simulink model "LQR_control"  (R2020b)
settings: Solver=VariableStepAuto  StartTime=0.0  StopTime=180  RelTol=1e-3
values from neighbouring files (symbols this model uses):
  A_m = [0 1 0; M_alpha 0 M_alpha/V; -(F+N_alpha)/m 0 -N_alpha/(m*V)]    [state_space.m]
  B_m = [0;M_delta;Tc/m]    [state_space.m]
  C_m = diag([1 1 1])    [state_space.m]
  D_m = [0;0;0]    [state_space.m]
  K_1 = K(1)    [state_space.m]
  K_2 = K(2)    [state_space.m]
  K_3 = K(3)    [state_space.m]
  m = 38901    [state_space.m]
undefined symbols (not defined in the file or in its folder): Earth, WGS84
libraries: aerolibtransform2 x1, aerolibfltsims x1
settings Model: Creator=surya  LastModifiedBy=surya

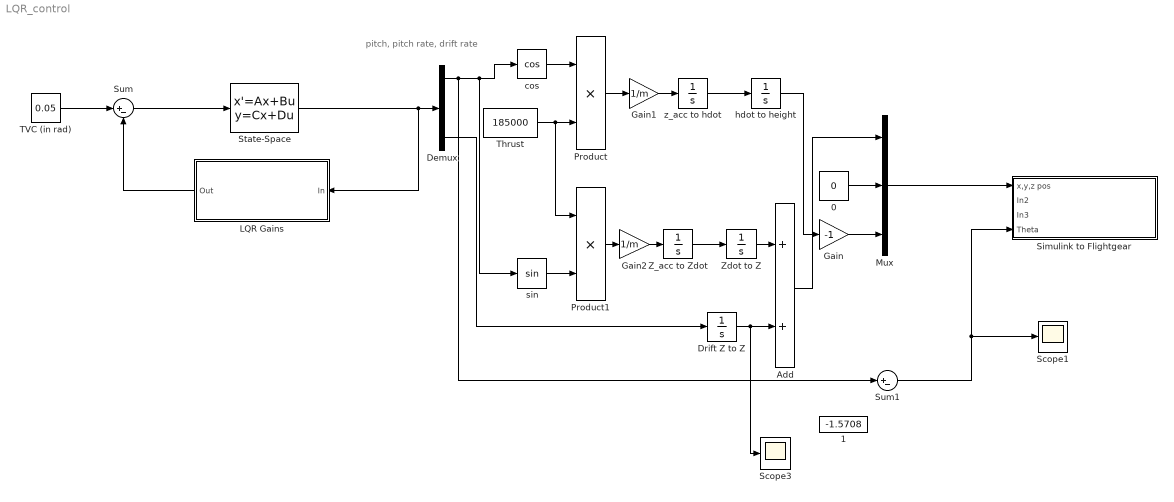
== system LQR_control ==
  note: pitch, pitch rate, drift rate
  0 : Constant  Value=0
  1 : Constant  Value=-1.5708
  Add : Sum
  Demux : Demux  Outputs=3
  Drift Z to Z : Integrator
  Gain : Gain  Gain=-1
  Gain1 : Gain  Gain=1/m
  Gain2 : Gain  Gain=1/m
  LQR Gains : Subsystem
  Mux : Mux  Inputs=3
  Product : Product
  Product1 : Product
  Scope1 : Scope
  Scope3 : Scope
  "Simulink to Flightgear " : Subsystem
  State-Space : StateSpace  A=A_m  B=B_m  C=C_m  D=D_m  InitialCondition=[0.2;0;0]
  Sum : Sum  Inputs=|+-
  Sum1 : Sum  Inputs=|+-
  TVC (in rad) : Constant  Value=0.05
  Thrust : Constant  Value=185000
  Z_acc to Zdot : Integrator
  Zdot to Z : Integrator
  cos : Trigonometry  Operator=cos
  hdot to height : Integrator
  sin : Trigonometry
  z_acc to hdot : Integrator
  wires:
  TVC (in rad)/1 -> Sum/1
  State-Space/1 -> LQR Gains/1(In), Demux/1
  Demux/1 -> Sum1/1, cos/1, sin/1
  cos/1 -> Product/1
  sin/1 -> Product1/2
  Thrust/1 -> Product1/1, Product/2
  Demux/3 -> Drift Z to Z/1
  Zdot to Z/1 -> Add/1
  Drift Z to Z/1 -> Scope3/1, Add/2
  hdot to height/1 -> Gain/1
  Add/1 -> Mux/1
  0/1 -> Mux/2
  Gain/1 -> Mux/3
  Sum1/1 -> Scope1/1, "Simulink to Flightgear "/4("Theta ")
  z_acc to hdot/1 -> hdot to height/1
  Z_acc to Zdot/1 -> Zdot to Z/1
  Mux/1 -> "Simulink to Flightgear "/1(x,y,z pos)
  Product/1 -> Gain1/1
  Gain1/1 -> z_acc to hdot/1
  Product1/1 -> Gain2/1
  Gain2/1 -> Z_acc to Zdot/1
  LQR Gains/1(Out) -> Sum/2
  Sum/1 -> State-Space/1

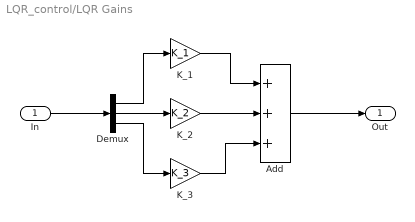
== system LQR_control/LQR Gains ==
  In : Inport
  Add : Sum  Inputs=+++
  Demux : Demux  Outputs=3
  K_1 : Gain  Gain=K_1
  K_2 : Gain  Gain=K_2
  K_3 : Gain  Gain=K_3
  Out : Outport
  wires:
  In/1 -> Demux/1
  K_3/1 -> Add/3
  K_1/1 -> Add/1
  Demux/3 -> K_3/1
  K_2/1 -> Add/2
  Demux/2 -> K_2/1
  Demux/1 -> K_1/1
  Add/1 -> Out/1

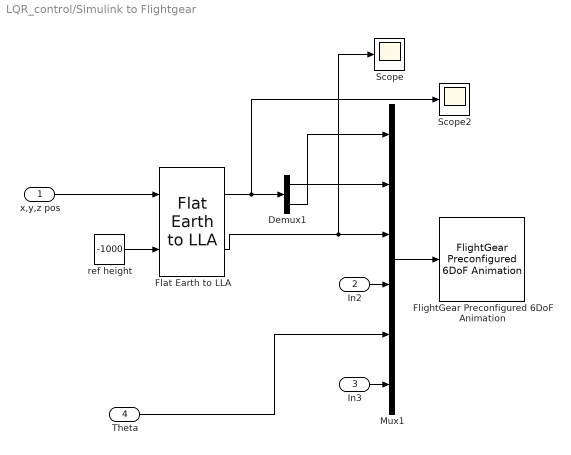
== system LQR_control/Simulink to Flightgear  ==
  x,y,z pos : Inport
  In2 : Inport  Port=2
  In3 : Inport  Port=3
  "Theta " : Inport  Port=4
  Demux1 : Demux  Outputs=2
  Flat Earth to LLA : aerolibtransform2/Flat Earth to LLA  units=Metric (MKS)  ptype=Earth (WGS84)  F=1/298.257223563  R=6378137  refPosPort=off  LL0=[34.9100 -117.8912]  psi=0
  FlightGear Preconfigured 6DoF Animation : aerolibfltsims/FlightGear Preconfigured 6DoF Animation  xFlightGearVersion=v2019.1  DestinationIpAddress=127.0.0.1  DestinationPort=5502  SampleTime=1/30  packetVersion=24
  Mux1 : Mux  Inputs=6
  Scope : Scope
  Scope2 : Scope
  ref height : Constant  Value=-1000
  wires:
  Flat Earth to LLA/2 -> Scope/1, Mux1/3
  Flat Earth to LLA/1 -> Scope2/1, Demux1/1
  ref height/1 -> Flat Earth to LLA/2
  Demux1/1 -> Mux1/2
  Mux1/1 -> FlightGear Preconfigured 6DoF Animation/1
  Demux1/2 -> Mux1/1
  In2/1 -> Mux1/4
  x,y,z pos/1 -> Flat Earth to LLA/1
  In3/1 -> Mux1/6
  "Theta "/1 -> Mux1/5
